simulink model "switching_leg"  (R2018a)
settings: Solver=FixedStepAuto  StartTime=0.0  StopTime=0.04  FixedStep=2.5e-6  RelTol=1e-3
libraries: powerlib_meascontrol x12
settings Model: Creator=enes_  LastModifiedBy=enes_

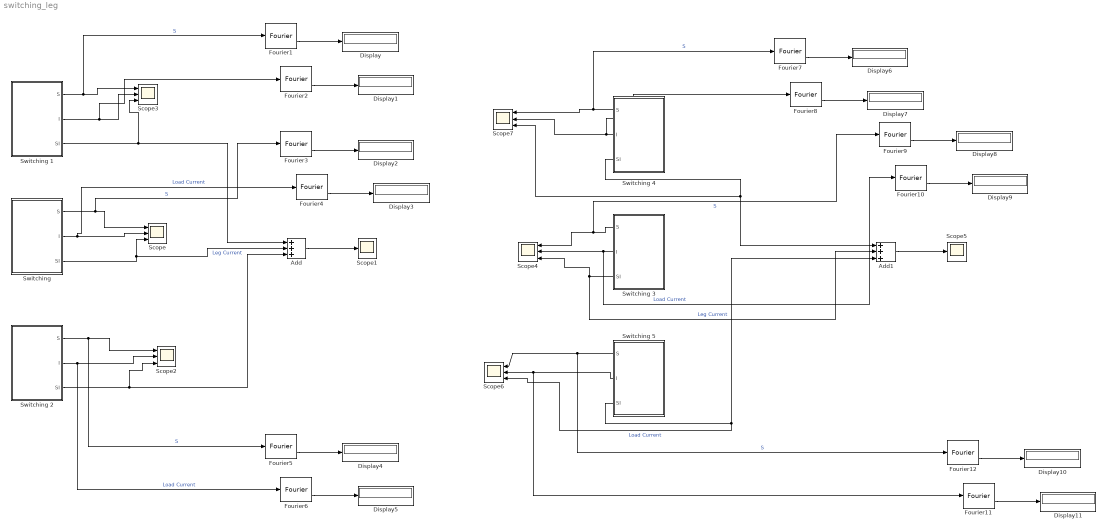
== system switching_leg ==
  Add : Sum  Inputs=3
  Add1 : Sum  Inputs=3
  Display{,1..11} (12 alike) : Display
  Fourier{1..12} (12 alike) : powerlib_meascontrol/Measurements/Fourier  Freq=50  n=1  InInit=[0, 0]  Ts=0
      settings: SourceProductName=Simscape Power Systems
  Scope{,2..4,6..7} (6 alike) : Scope  NumInputPorts=3
  Scope1 : Scope
  Scope5 : Scope
  "Switching " : Subsystem  mask{m=0.9, f_s=4e4, f_f=50, the_f=2*pi/3, the_c=0, i1=40, i2=40, load_phase=pi/6}
      mask prompts: m "modulation index"; f_s "carrier frequency"; f_f "fundemental frequency"; the_f "phase of fundamental"; the_c "phase of carrier"; i1 "iteration number of carrier"; i2 "iteration number of fundamental"; load_phase "phase of load current"
  Switching 1 : Subsystem  mask{m=0.9, f_s=4e4, f_f=50, the_f=0, the_c=0, i1=40, i2=40, load_phase=pi/6}
      mask prompts: m "modulation index"; f_s "carrier frequency"; f_f "fundemental frequency"; the_f "phase of fundamental"; the_c "phase of carrier"; i1 "iteration number of carrier"; i2 "iteration number of fundamental"; load_phase "phase of load current"
  Switching 2 : Subsystem  mask{m=0.9, f_s=4e4, f_f=50, the_f=4*pi/3, the_c=0, i1=40, i2=40, load_phase=pi/6}
      mask prompts: m "modulation index"; f_s "carrier frequency"; f_f "fundemental frequency"; the_f "phase of fundamental"; the_c "phase of carrier"; i1 "iteration number of carrier"; i2 "iteration number of fundamental"; load_phase "phase of load current"
  Switching 3 : Subsystem  mask{m=0.9, f_s=4e4, f_f=50, the_f=2*pi/3, the_c=3*pi/4, i1=40, i2=40, load_phase=pi/6}
      mask prompts: m "modulation index"; f_s "carrier frequency"; f_f "fundemental frequency"; the_f "phase of fundamental"; the_c "phase of carrier"; i1 "iteration number of carrier"; i2 "iteration number of fundamental"; load_phase "phase of load current"
  Switching 4 : Subsystem  mask{m=0.9, f_s=4e4, f_f=50, the_f=0, the_c=3*pi/4, i1=40, i2=40, load_phase=pi/6}
      mask prompts: m "modulation index"; f_s "carrier frequency"; f_f "fundemental frequency"; the_f "phase of fundamental"; the_c "phase of carrier"; i1 "iteration number of carrier"; i2 "iteration number of fundamental"; load_phase "phase of load current"
  Switching 5 : Subsystem  mask{m=0.9, f_s=4e4, f_f=50, the_f=4*pi/3, the_c=3*pi/4, i1=40, i2=40, load_phase=pi/6}
      mask prompts: m "modulation index"; f_s "carrier frequency"; f_f "fundemental frequency"; the_f "phase of fundamental"; the_c "phase of carrier"; i1 "iteration number of carrier"; i2 "iteration number of fundamental"; load_phase "phase of load current"
  wires:
  "Switching "/2("I ") -> Fourier4/1, Scope/2  "Load Current"
  "Switching "/3(SI) -> Add/2, Scope/3  "Leg Current"
  Switching 1/3(SI) -> Scope3/3, Add/1
  Switching 2/3(SI) -> Scope2/3, Add/3
  Add/1 -> Scope1/1
  Switching 3/3(SI) -> Scope4/3, Add1/2  "Leg Current"
  Add1/1 -> Scope5/1
  Switching 5/2("I ") -> Fourier11/1, Scope6/2
  Switching 4/3(SI) -> Add1/1, Scope7/3
  Fourier1/2 -> Display/1
  Switching 1/1(S) -> Fourier1/1, Scope3/1  "S"
  Fourier2/2 -> Display1/1
  Switching 1/2("I ") -> Fourier2/1, Scope3/2
  "Switching "/1(S) -> Fourier3/1, Scope/1  "S"
  Fourier3/2 -> Display2/1
  Fourier4/2 -> Display3/1
  Fourier6/2 -> Display5/1
  Fourier5/2 -> Display4/1
  Switching 2/1(S) -> Fourier5/1, Scope2/1  "S"
  Switching 2/2("I ") -> Fourier6/1, Scope2/2  "Load Current"
  Switching 4/1(S) -> Fourier7/1, Scope7/1  "S"
  Switching 4/2("I ") -> Fourier8/1, Scope7/2
  Fourier7/2 -> Display6/1
  Fourier8/2 -> Display7/1
  Fourier10/2 -> Display9/1
  Fourier9/2 -> Display8/1
  Switching 3/1(S) -> Fourier9/1, Scope4/1  "S"
  Switching 3/2("I ") -> Fourier10/1, Scope4/2  "Load Current"
  Switching 5/3(SI) -> Add1/3, Scope6/3  "Load Current"
  Fourier12/2 -> Display10/1
  Fourier11/2 -> Display11/1
  Switching 5/1(S) -> Fourier12/1, Scope6/1  "S"

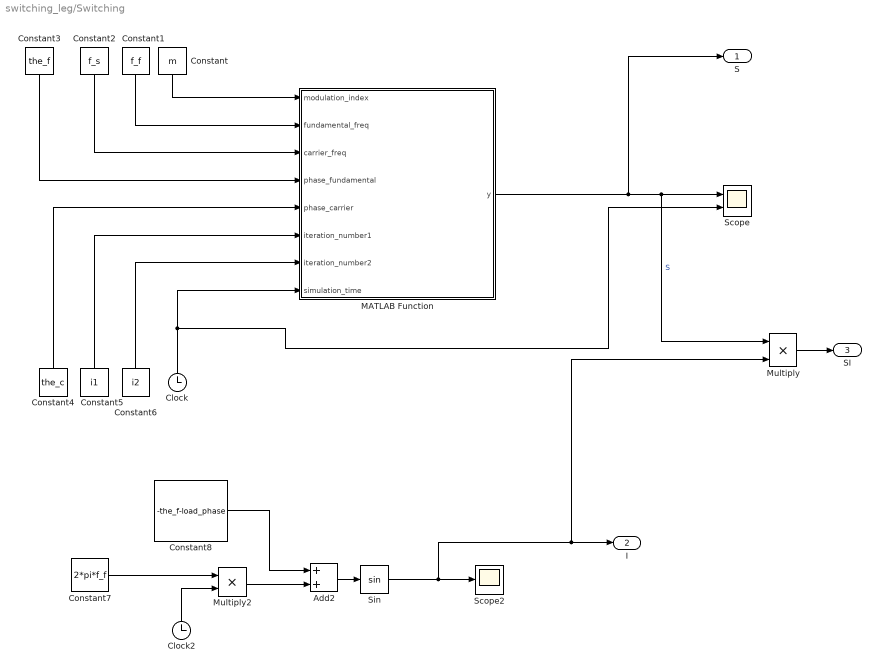
== system switching_leg/Switching  ==
  Add2 : Sum
  Clock : Clock
  Clock2 : Clock
  Constant : Constant  Value=m
  Constant1 : Constant  Value=f_f
  Constant2 : Constant  Value=f_s
  Constant3 : Constant  Value=the_f
  Constant4 : Constant  Value=the_c
  Constant5 : Constant  Value=i1
  Constant6 : Constant  Value=i2
  Constant7 : Constant  Value=2*pi*f_f
  Constant8 : Constant  Value=-the_f-load_phase  VectorParams1D=off
  MATLAB Function : MATLAB Function  TreatAsAtomicUnit=on
  Multiply : Product
  Multiply2 : Product
  Scope : Scope  NumInputPorts=2
  Scope2 : Scope
  Sin : Trigonometry
  S : Outport
  "I " : Outport  Port=2
  SI : Outport  Port=3
  wires:
  Constant/1 -> MATLAB Function/1(modulation_index)
  Constant1/1 -> MATLAB Function/2(fundamental_freq)
  Constant2/1 -> MATLAB Function/3(carrier_freq)
  Constant3/1 -> MATLAB Function/4(phase_fundamental)
  Constant4/1 -> MATLAB Function/5(phase_carrier)
  Constant5/1 -> MATLAB Function/6(iteration_number1)
  Constant6/1 -> MATLAB Function/7(iteration_number2)
  MATLAB Function/1(y) -> S/1, Multiply/1, Scope/1  "S"
  Clock/1 -> Scope/2, MATLAB Function/8(simulation_time)
  Constant7/1 -> Multiply2/1
  Sin/1 -> Multiply/2, "I "/1, Scope2/1
  Add2/1 -> Sin/1
  Clock2/1 -> Multiply2/2
  Constant8/1 -> Add2/1
  Multiply2/1 -> Add2/2
  Multiply/1 -> SI/1

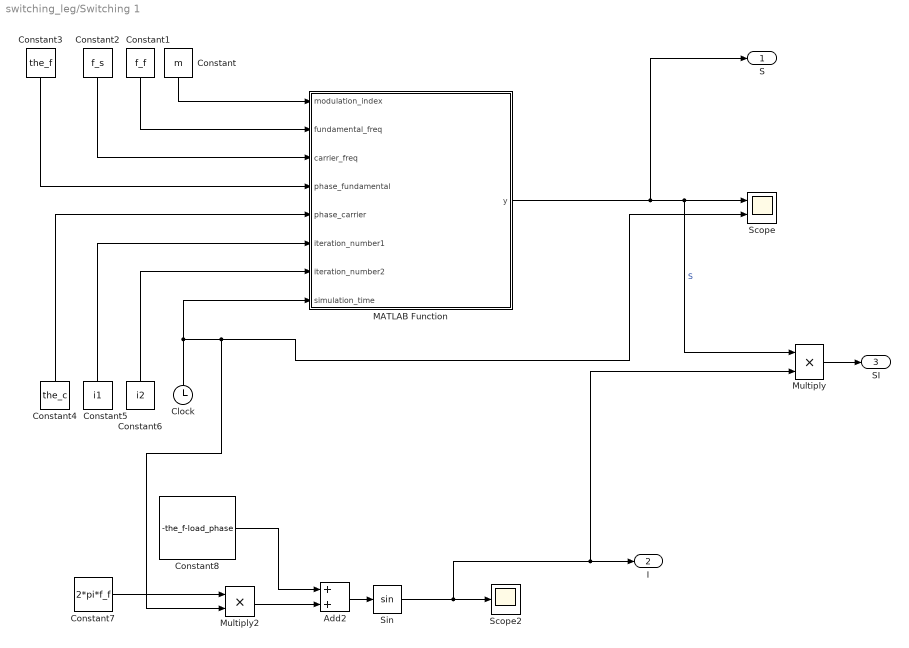
== system switching_leg/Switching 1 ==
  Add2 : Sum
  Clock : Clock
  Constant : Constant  Value=m
  Constant1 : Constant  Value=f_f
  Constant2 : Constant  Value=f_s
  Constant3 : Constant  Value=the_f
  Constant4 : Constant  Value=the_c
  Constant5 : Constant  Value=i1
  Constant6 : Constant  Value=i2
  Constant7 : Constant  Value=2*pi*f_f
  Constant8 : Constant  Value=-the_f-load_phase  VectorParams1D=off
  MATLAB Function : MATLAB Function  TreatAsAtomicUnit=on
  Multiply : Product
  Multiply2 : Product
  Scope : Scope  NumInputPorts=2
  Scope2 : Scope
  Sin : Trigonometry
  S : Outport
  "I " : Outport  Port=2
  SI : Outport  Port=3
  wires:
  Constant/1 -> MATLAB Function/1(modulation_index)
  Constant1/1 -> MATLAB Function/2(fundamental_freq)
  Constant2/1 -> MATLAB Function/3(carrier_freq)
  Constant3/1 -> MATLAB Function/4(phase_fundamental)
  Constant4/1 -> MATLAB Function/5(phase_carrier)
  Constant5/1 -> MATLAB Function/6(iteration_number1)
  Constant6/1 -> MATLAB Function/7(iteration_number2)
  MATLAB Function/1(y) -> S/1, Multiply/1, Scope/1  "S"
  Constant7/1 -> Multiply2/1
  Sin/1 -> Multiply/2, "I "/1, Scope2/1
  Add2/1 -> Sin/1
  Clock/1 -> Multiply2/2, Scope/2, MATLAB Function/8(simulation_time)
  Constant8/1 -> Add2/1
  Multiply2/1 -> Add2/2
  Multiply/1 -> SI/1

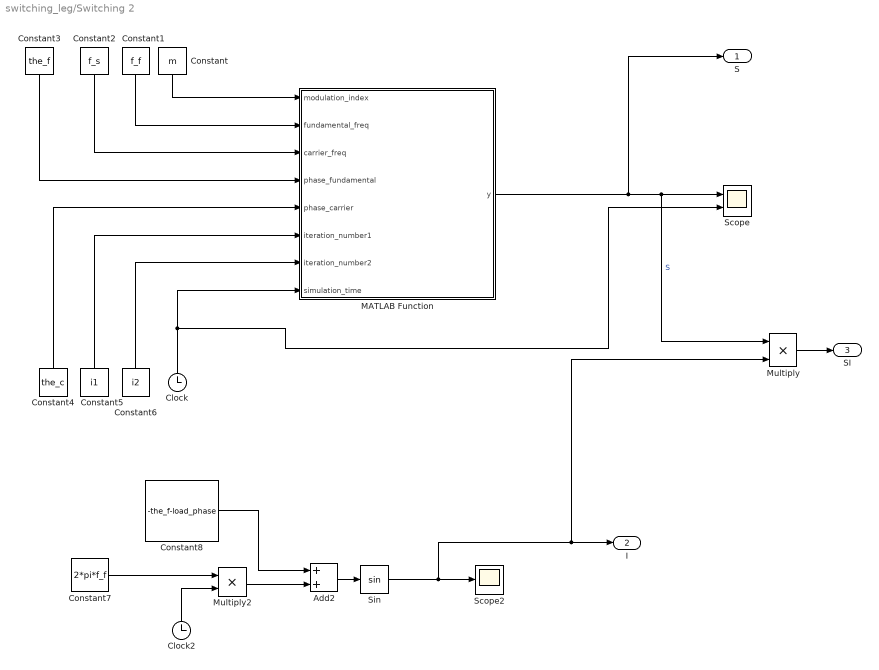
== system switching_leg/Switching 2 ==
  Add2 : Sum
  Clock : Clock
  Clock2 : Clock
  Constant : Constant  Value=m
  Constant1 : Constant  Value=f_f
  Constant2 : Constant  Value=f_s
  Constant3 : Constant  Value=the_f
  Constant4 : Constant  Value=the_c
  Constant5 : Constant  Value=i1
  Constant6 : Constant  Value=i2
  Constant7 : Constant  Value=2*pi*f_f
  Constant8 : Constant  Value=-the_f-load_phase  VectorParams1D=off
  MATLAB Function : MATLAB Function  TreatAsAtomicUnit=on
  Multiply : Product
  Multiply2 : Product
  Scope : Scope  NumInputPorts=2
  Scope2 : Scope
  Sin : Trigonometry
  S : Outport
  "I " : Outport  Port=2
  SI : Outport  Port=3
  wires:
  Constant/1 -> MATLAB Function/1(modulation_index)
  Constant1/1 -> MATLAB Function/2(fundamental_freq)
  Constant2/1 -> MATLAB Function/3(carrier_freq)
  Constant3/1 -> MATLAB Function/4(phase_fundamental)
  Constant4/1 -> MATLAB Function/5(phase_carrier)
  Constant5/1 -> MATLAB Function/6(iteration_number1)
  Constant6/1 -> MATLAB Function/7(iteration_number2)
  MATLAB Function/1(y) -> S/1, Multiply/1, Scope/1  "S"
  Clock/1 -> Scope/2, MATLAB Function/8(simulation_time)
  Constant7/1 -> Multiply2/1
  Sin/1 -> Multiply/2, "I "/1, Scope2/1
  Add2/1 -> Sin/1
  Clock2/1 -> Multiply2/2
  Constant8/1 -> Add2/1
  Multiply2/1 -> Add2/2
  Multiply/1 -> SI/1

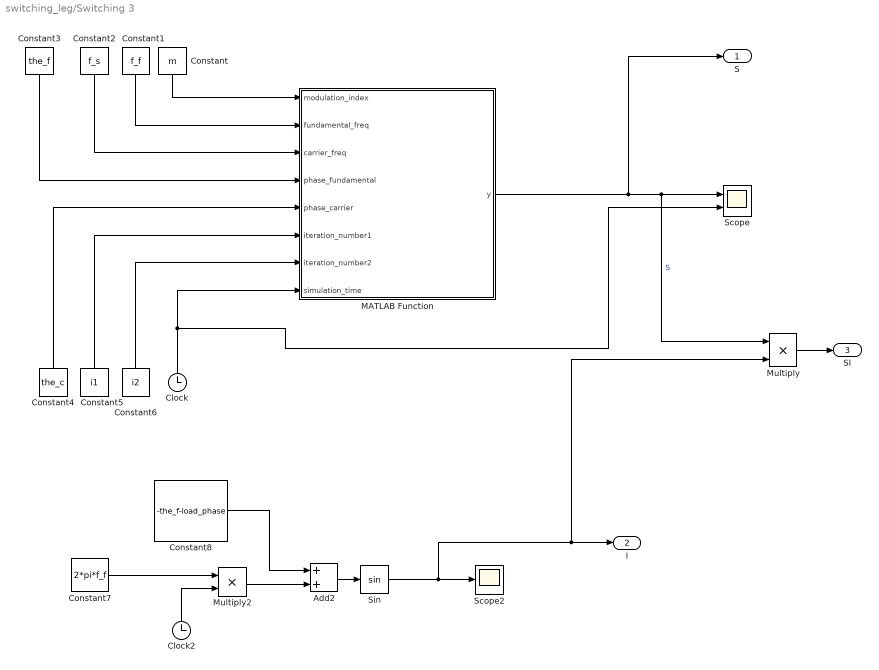
== system switching_leg/Switching 3 ==
  Add2 : Sum
  Clock : Clock
  Clock2 : Clock
  Constant : Constant  Value=m
  Constant1 : Constant  Value=f_f
  Constant2 : Constant  Value=f_s
  Constant3 : Constant  Value=the_f
  Constant4 : Constant  Value=the_c
  Constant5 : Constant  Value=i1
  Constant6 : Constant  Value=i2
  Constant7 : Constant  Value=2*pi*f_f
  Constant8 : Constant  Value=-the_f-load_phase
  MATLAB Function : MATLAB Function  TreatAsAtomicUnit=on
  Multiply : Product
  Multiply2 : Product
  Scope : Scope  NumInputPorts=2
  Scope2 : Scope
  Sin : Trigonometry
  S : Outport
  "I " : Outport  Port=2
  SI : Outport  Port=3
  wires:
  Constant/1 -> MATLAB Function/1(modulation_index)
  Constant1/1 -> MATLAB Function/2(fundamental_freq)
  Constant2/1 -> MATLAB Function/3(carrier_freq)
  Constant3/1 -> MATLAB Function/4(phase_fundamental)
  Constant4/1 -> MATLAB Function/5(phase_carrier)
  Constant5/1 -> MATLAB Function/6(iteration_number1)
  Constant6/1 -> MATLAB Function/7(iteration_number2)
  MATLAB Function/1(y) -> S/1, Multiply/1, Scope/1  "S"
  Clock/1 -> Scope/2, MATLAB Function/8(simulation_time)
  Constant7/1 -> Multiply2/1
  Sin/1 -> Multiply/2, "I "/1, Scope2/1
  Add2/1 -> Sin/1
  Clock2/1 -> Multiply2/2
  Constant8/1 -> Add2/1
  Multiply2/1 -> Add2/2
  Multiply/1 -> SI/1

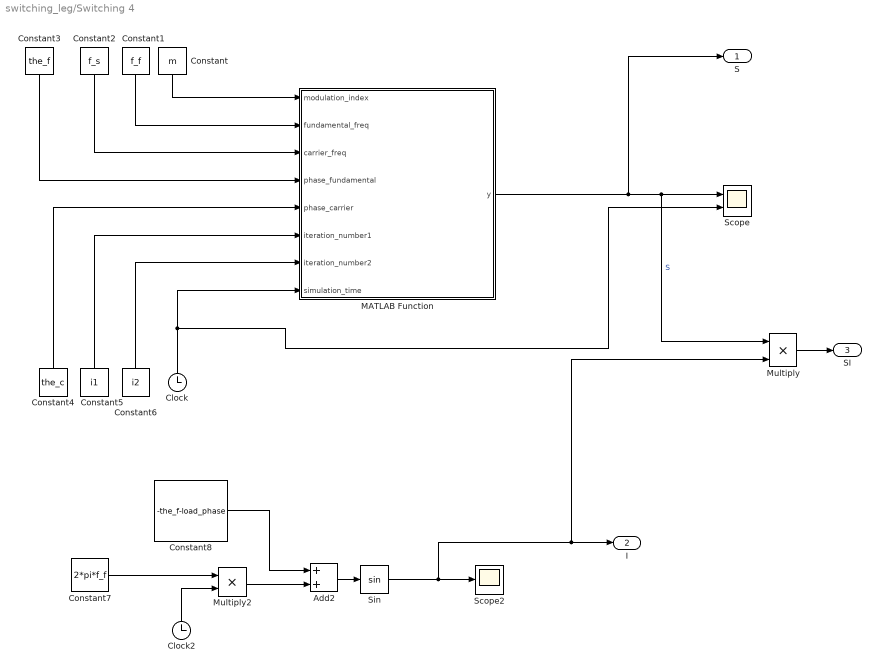
== system switching_leg/Switching 4 ==
  Add2 : Sum
  Clock : Clock
  Clock2 : Clock
  Constant : Constant  Value=m
  Constant1 : Constant  Value=f_f
  Constant2 : Constant  Value=f_s
  Constant3 : Constant  Value=the_f
  Constant4 : Constant  Value=the_c
  Constant5 : Constant  Value=i1
  Constant6 : Constant  Value=i2
  Constant7 : Constant  Value=2*pi*f_f
  Constant8 : Constant  Value=-the_f-load_phase
  MATLAB Function : MATLAB Function  TreatAsAtomicUnit=on
  Multiply : Product
  Multiply2 : Product
  Scope : Scope  NumInputPorts=2
  Scope2 : Scope
  Sin : Trigonometry
  S : Outport
  "I " : Outport  Port=2
  SI : Outport  Port=3
  wires:
  Constant/1 -> MATLAB Function/1(modulation_index)
  Constant1/1 -> MATLAB Function/2(fundamental_freq)
  Constant2/1 -> MATLAB Function/3(carrier_freq)
  Constant3/1 -> MATLAB Function/4(phase_fundamental)
  Constant4/1 -> MATLAB Function/5(phase_carrier)
  Constant5/1 -> MATLAB Function/6(iteration_number1)
  Constant6/1 -> MATLAB Function/7(iteration_number2)
  MATLAB Function/1(y) -> S/1, Multiply/1, Scope/1  "S"
  Clock/1 -> Scope/2, MATLAB Function/8(simulation_time)
  Constant7/1 -> Multiply2/1
  Sin/1 -> Multiply/2, "I "/1, Scope2/1
  Add2/1 -> Sin/1
  Clock2/1 -> Multiply2/2
  Constant8/1 -> Add2/1
  Multiply2/1 -> Add2/2
  Multiply/1 -> SI/1

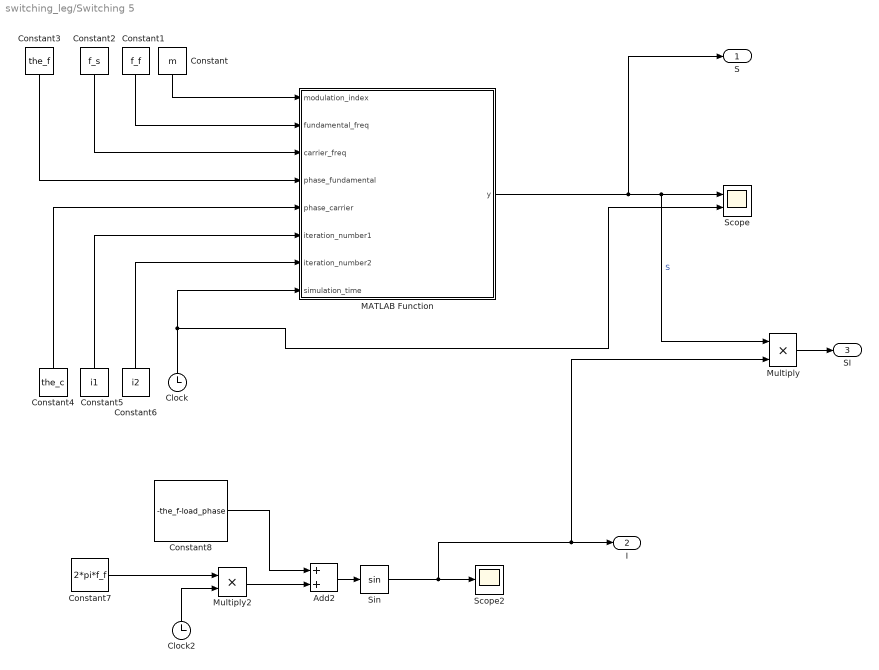
== system switching_leg/Switching 5 ==
  Add2 : Sum
  Clock : Clock
  Clock2 : Clock
  Constant : Constant  Value=m
  Constant1 : Constant  Value=f_f
  Constant2 : Constant  Value=f_s
  Constant3 : Constant  Value=the_f
  Constant4 : Constant  Value=the_c
  Constant5 : Constant  Value=i1
  Constant6 : Constant  Value=i2
  Constant7 : Constant  Value=2*pi*f_f
  Constant8 : Constant  Value=-the_f-load_phase
  MATLAB Function : MATLAB Function  TreatAsAtomicUnit=on
  Multiply : Product
  Multiply2 : Product
  Scope : Scope  NumInputPorts=2
  Scope2 : Scope
  Sin : Trigonometry
  S : Outport
  "I " : Outport  Port=2
  SI : Outport  Port=3
  wires:
  Constant/1 -> MATLAB Function/1(modulation_index)
  Constant1/1 -> MATLAB Function/2(fundamental_freq)
  Constant2/1 -> MATLAB Function/3(carrier_freq)
  Constant3/1 -> MATLAB Function/4(phase_fundamental)
  Constant4/1 -> MATLAB Function/5(phase_carrier)
  Constant5/1 -> MATLAB Function/6(iteration_number1)
  Constant6/1 -> MATLAB Function/7(iteration_number2)
  MATLAB Function/1(y) -> S/1, Multiply/1, Scope/1  "S"
  Clock/1 -> Scope/2, MATLAB Function/8(simulation_time)
  Constant7/1 -> Multiply2/1
  Sin/1 -> Multiply/2, "I "/1, Scope2/1
  Add2/1 -> Sin/1
  Clock2/1 -> Multiply2/2
  Constant8/1 -> Add2/1
  Multiply2/1 -> Add2/2
  Multiply/1 -> SI/1

== matlab function switching_leg/Switching 1/MATLAB Function ==
  data: modulation_index input; y output; fundamental_freq input; carrier_freq input; phase_fundamental input; phase_carrier input; iteration_number1 input; iteration_number2 input; simulation_time input
function y  = fcn(modulation_index, fundamental_freq,carrier_freq,phase_fundamental, phase_carrier, iteration_number1,iteration_number2,simulation_time)

y=0;

fundamental_angFreq=2*pi*fundamental_freq;
carrier_angFreq= 2*pi*carrier_freq;
phase_fundamental=phase_fundamental+pi/2;


for m=1:iteration_number1
    for n= -iteration_number2:iteration_number2  
        k=(2/(m*pi))*sin((m+n)*pi/2)*...
                besselj(n,m*modulation_index*pi/2)*...
                cos(m*(carrier_angFreq*simulation_time-phase_carrier)...
                +n*(fundamental_angFreq*simulation_time-phase_fundamental));
       y=y+real(k);
          
        
        
    end
end

y= y+(1/2)+ (modulation_index/2)*cos(fundamental_angFreq*simulation_time-phase_fundamental);

== matlab function switching_leg/Switching 2/MATLAB Function ==
  data: modulation_index input; y output; fundamental_freq input; carrier_freq input; phase_fundamental input; phase_carrier input; iteration_number1 input; iteration_number2 input; simulation_time input
function y  = fcn(modulation_index, fundamental_freq,carrier_freq,phase_fundamental, phase_carrier, iteration_number1,iteration_number2,simulation_time)

y=0;

fundamental_angFreq=2*pi*fundamental_freq;
carrier_angFreq= 2*pi*carrier_freq;
phase_fundamental=phase_fundamental+pi/2;


for m=1:iteration_number1
    for n= -iteration_number2:iteration_number2  
        k=(2/(m*pi))*sin((m+n)*pi/2)*...
                besselj(n,m*modulation_index*pi/2)*...
                cos(m*(carrier_angFreq*simulation_time-phase_carrier)...
                +n*(fundamental_angFreq*simulation_time-phase_fundamental));
       y=y+real(k);
          
        
        
    end
end

y= y+(1/2)+ (modulation_index/2)*cos(fundamental_angFreq*simulation_time-phase_fundamental);

== matlab function switching_leg/Switching 3/MATLAB Function ==
  data: modulation_index input; y output; fundamental_freq input; carrier_freq input; phase_fundamental input; phase_carrier input; iteration_number1 input; iteration_number2 input; simulation_time input
function y  = fcn(modulation_index, fundamental_freq,carrier_freq,phase_fundamental, phase_carrier, iteration_number1,iteration_number2,simulation_time)

y=0;

fundamental_angFreq=2*pi*fundamental_freq;
carrier_angFreq= 2*pi*carrier_freq;
phase_fundamental=phase_fundamental+pi/2;


for m=1:iteration_number1
    for n= -iteration_number2:iteration_number2  
        k=(2/(m*pi))*sin((m+n)*pi/2)*...
                besselj(n,m*modulation_index*pi/2)*...
                cos(m*(carrier_angFreq*simulation_time-phase_carrier)...
                +n*(fundamental_angFreq*simulation_time-phase_fundamental));
       y=y+real(k);
          
        
        
    end
end

y= y+(1/2)+ (modulation_index/2)*cos(fundamental_angFreq*simulation_time-phase_fundamental);

== matlab function switching_leg/Switching /MATLAB Function ==
  data: modulation_index input; y output; fundamental_freq input; carrier_freq input; phase_fundamental input; phase_carrier input; iteration_number1 input; iteration_number2 input; simulation_time input
function y  = fcn(modulation_index, fundamental_freq,carrier_freq,phase_fundamental, phase_carrier, iteration_number1,iteration_number2,simulation_time)

y=0;

fundamental_angFreq=2*pi*fundamental_freq;
carrier_angFreq= 2*pi*carrier_freq;
phase_fundamental=phase_fundamental+pi/2;


for m=1:iteration_number1
    for n= -iteration_number2:iteration_number2  
        k=(2/(m*pi))*sin((m+n)*pi/2)*...
                besselj(n,m*modulation_index*pi/2)*...
                cos(m*(carrier_angFreq*simulation_time-phase_carrier)...
                +n*(fundamental_angFreq*simulation_time-phase_fundamental));
       y=y+real(k);
          
        
        
    end
end

y= y+(1/2)+ (modulation_index/2)*cos(fundamental_angFreq*simulation_time-phase_fundamental);

== matlab function switching_leg/Switching 4/MATLAB Function ==
  data: modulation_index input; y output; fundamental_freq input; carrier_freq input; phase_fundamental input; phase_carrier input; iteration_number1 input; iteration_number2 input; simulation_time input
function y  = fcn(modulation_index, fundamental_freq,carrier_freq,phase_fundamental, phase_carrier, iteration_number1,iteration_number2,simulation_time)

y=0;

fundamental_angFreq=2*pi*fundamental_freq;
carrier_angFreq= 2*pi*carrier_freq;
phase_fundamental=phase_fundamental+pi/2;


for m=1:iteration_number1
    for n= -iteration_number2:iteration_number2  
        k=(2/(m*pi))*sin((m+n)*pi/2)*...
                besselj(n,m*modulation_index*pi/2)*...
                cos(m*(carrier_angFreq*simulation_time-phase_carrier)...
                +n*(fundamental_angFreq*simulation_time-phase_fundamental));
       y=y+real(k);
          
        
        
    end
end

y= y+(1/2)+ (modulation_index/2)*cos(fundamental_angFreq*simulation_time-phase_fundamental);

== matlab function switching_leg/Switching 5/MATLAB Function ==
  data: modulation_index input; y output; fundamental_freq input; carrier_freq input; phase_fundamental input; phase_carrier input; iteration_number1 input; iteration_number2 input; simulation_time input
function y  = fcn(modulation_index, fundamental_freq,carrier_freq,phase_fundamental, phase_carrier, iteration_number1,iteration_number2,simulation_time)

y=0;

fundamental_angFreq=2*pi*fundamental_freq;
carrier_angFreq= 2*pi*carrier_freq;
phase_fundamental=phase_fundamental+pi/2;


for m=1:iteration_number1
    for n= -iteration_number2:iteration_number2  
        k=(2/(m*pi))*sin((m+n)*pi/2)*...
                besselj(n,m*modulation_index*pi/2)*...
                cos(m*(carrier_angFreq*simulation_time-phase_carrier)...
                +n*(fundamental_angFreq*simulation_time-phase_fundamental));
       y=y+real(k);
          
        
        
    end
end

y= y+(1/2)+ (modulation_index/2)*cos(fundamental_angFreq*simulation_time-phase_fundamental);
